simulink library "SUB_ECU_Transmission"  (R2018a)
settings: Solver=VariableStepAuto  StartTime=0.0  StopTime=10.0  RelTol=1e-3
libraries: PTC_MBDS_LIB x38, simulink x9
settings Model: Creator=Sundeep.Tuteja  LastModifiedBy=John.Lahti

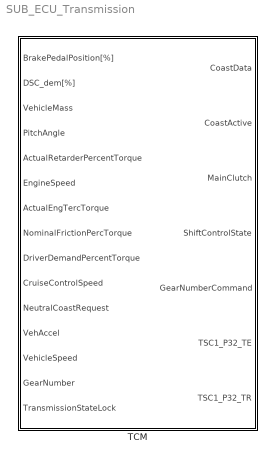
== system SUB_ECU_Transmission ==
  TCM : Subsystem  TreatAsAtomicUnit=on  SystemSampleTime=.01

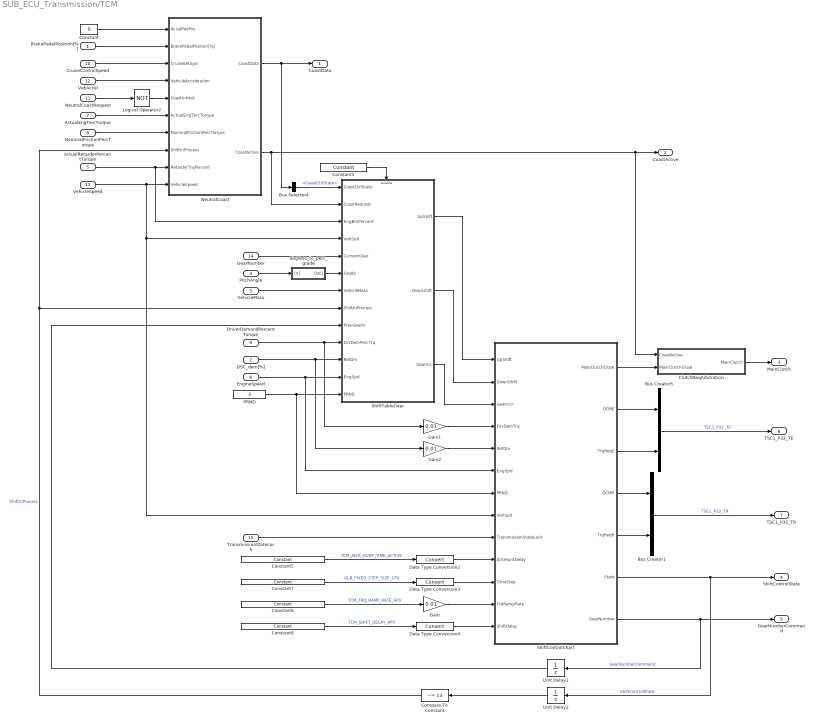
== system SUB_ECU_Transmission/TCM ==
  BrakePedalPosition[%] : Inport  Unit=%
  DSC_dem[%] : Inport  Port=2  Unit=%
  VehicleMass : Inport  Port=3
  PitchAngle : Inport  Port=4
  ActualRetarderPercentTorque : Inport  Port=5
  EngineSpeed : Inport  Port=6
  ActualEngTercTorque : Inport  Port=7
  NominalFrictionPercTorque : Inport  Port=8
  DriverDemandPercentTorque : Inport  Port=9
  CruiseControlSpeed : Inport  Port=10  Unit=km/h
  NeutralCoastRequest : Inport  Port=11
  VehAccel : Inport  Port=12
  VehicleSpeed : Inport  Port=13
  GearNumber : Inport  Port=14
  TransmissionStateLock : Inport  Port=15
  Bus Creator1 : BusCreator  Inputs=2
  Bus Creator5 : BusCreator  Inputs=2
  Bus Selector4 : BusSelector  OutputSignals=CoastCtrlState
  ClutchReqArbitration : Subsystem
  Compare To Constant : simulink/Logic and Bit Operations/Compare To Constant  relop=~=  const=13  OutDataTypeStr=boolean
  Constant : Constant  Value=0
  Constant3 : PTC_MBDS_LIB/Extras/Sources/Constant  Value2=true  PTC_MBDS_BlockVersion=5.41  PTC_BlockType=PTC_MBDS_Constant
      settings: SourceProductName=PACCAR Technical Center MBDS Library
  Constant5 : PTC_MBDS_LIB/Extras/Sources/Constant  Value2=TCM_ANTI_HUNT_TIME_ACTIVE  PTC_MBDS_BlockVersion=5.41  PTC_BlockType=PTC_MBDS_Constant
      settings: SourceProductName=PACCAR Technical Center MBDS Library
      settings: AttributesFormatString=|
      | Value: 1
      | Unit: 's'
  Constant6 : PTC_MBDS_LIB/Extras/Sources/Constant  Value2=TCM_TRQ_RAMP_RATE_APV  PTC_MBDS_BlockVersion=5.41  PTC_BlockType=PTC_MBDS_Constant
      settings: SourceProductName=PACCAR Technical Center MBDS Library
      settings: AttributesFormatString=|
      | Value: 121
      | Unit: '%/s'
  Constant7 : PTC_MBDS_LIB/Extras/Sources/Constant  Value2=GLB_FIXED_STEP_SIZE_CPV  PTC_MBDS_BlockVersion=5.41  PTC_BlockType=PTC_MBDS_Constant
      settings: SourceProductName=PACCAR Technical Center MBDS Library
      settings: AttributesFormatString=|
      | Value: 0.01
      | Unit: 's'
  Constant8 : PTC_MBDS_LIB/Extras/Sources/Constant  Value2=TCM_SHIFT_DELAY_APV  PTC_MBDS_BlockVersion=5.41  PTC_BlockType=PTC_MBDS_Constant
      settings: SourceProductName=PACCAR Technical Center MBDS Library
      settings: AttributesFormatString=|
      | Value: 0.949999988079
      | Unit: 's'
  Data Type Conversion2 : DataTypeConversion  SaturateOnIntegerOverflow=on
  Data Type Conversion3 : DataTypeConversion  SaturateOnIntegerOverflow=on
  Data Type Conversion4 : DataTypeConversion  SaturateOnIntegerOverflow=on
  Gain : Gain  Gain=0.01
  Gain1 : Gain  Gain=0.01
  Gain2 : Gain  Gain=0.01
  Logical Operator2 : Logic  Operator=NOT  AllPortsSameDT=off  OutDataTypeStr=boolean
  NeutralCoast : Subsystem
  PRND : Constant  Value=3
  ShiftControlChart : Stateflow chart  TreatAsAtomicUnit=on
      settings: MinAlgLoopOccurrences=on
  ShiftTableGear : Subsystem
  Unit Delay1 : UnitDelay  SampleTime=-1
  Unit Delay2 : UnitDelay  SampleTime=-1
  degrees_to_perc_grade : Subsystem
  CoastData : Outport
  CoastActive : Outport  Port=2
  MainClutch : Outport  Port=3
  ShiftControlState : Outport  Port=4
  GearNumberCommand : Outport  Port=5
  TSC1_P32_TE : Outport  Port=6
  TSC1_P32_TR : Outport  Port=7
  wires:
  ShiftControlChart/6(State) -> Unit Delay2/1, ShiftControlState/1  "ShiftControlState"
  ShiftControlChart/7(GearNumber) -> Unit Delay1/1, GearNumberCommand/1  "GearNumberCommand"
  Data Type Conversion4/1 -> ShiftControlChart/13(ShiftDelay)
  Data Type Conversion3/1 -> ShiftControlChart/11(TimeStep)
  Data Type Conversion2/1 -> ShiftControlChart/10(AntiHuntDelay)
  VehicleMass/1 -> ShiftTableGear/7(VehicleMass)
  Gain/1 -> ShiftControlChart/12(TrqRampRate)
  Constant3/1 -> ShiftTableGear/Enable
  DSC_dem[%]/1 -> Gain2/1, ShiftTableGear/11(RetDrv)
  Constant8/1 -> Data Type Conversion4/1  "TCM_SHIFT_DELAY_APV"
  Constant6/1 -> Gain/1  "TCM_TRQ_RAMP_RATE_APV"
  VehAccel/1 -> NeutralCoast/4(VehicleAcceleration)
  NeutralCoast/2(CoastActive) -> CoastActive/1, ClutchReqArbitration/1(CoastActive), ShiftTableGear/2(CoastRequest)
  Bus Selector4/1 -> ShiftTableGear/1(CoastCtrlState)  "<CoastCtrlState>"
  ShiftControlChart/1(MainClutchClose) -> ClutchReqArbitration/2(MainClutchClose)
  CruiseControlSpeed/1 -> NeutralCoast/3(CruiseSetSpd)
  Constant5/1 -> Data Type Conversion2/1  "TCM_ANTI_HUNT_TIME_ACTIVE"
  Constant7/1 -> Data Type Conversion3/1  "GLB_FIXED_STEP_SIZE_CPV"
  ClutchReqArbitration/1(MainClutch) -> MainClutch/1
  Constant/1 -> NeutralCoast/1(AccelPedPos)
  VehicleSpeed/1 -> NeutralCoast/10(VehicleSpeed), ShiftControlChart/8(VehSpd), ShiftTableGear/4(VehSpd)
  EngineSpeed/1 -> ShiftTableGear/12(EngSpd), ShiftControlChart/6(EngSpd)
  degrees_to_perc_grade/1(Out1) -> ShiftTableGear/6(Grade)
  TransmissionStateLock/1 -> ShiftControlChart/9(TransmissionStateLock)
  ActualRetarderPercentTorque/1 -> ShiftTableGear/3(EngBrkPercent), NeutralCoast/9(RetarderTrqPercent)
  ActualEngTercTorque/1 -> NeutralCoast/6(ActualEngTercTorque)
  NominalFrictionPercTorque/1 -> NeutralCoast/7(NominalFrictionPercTorque)
  NeutralCoastRequest/1 -> Logical Operator2/1
  ShiftTableGear/1(UpShift) -> ShiftControlChart/1(UpShift)
  ShiftTableGear/2(Downshift) -> ShiftControlChart/2(DownShift)
  ShiftTableGear/3(GearInc) -> ShiftControlChart/3(GearIncr)
  Bus Creator5/1 -> TSC1_P32_TE/1  "TSC1_P32_TE"
  Bus Creator1/1 -> TSC1_P32_TR/1  "TSC1_P32_TR"
  Gain1/1 -> ShiftControlChart/4(DrvDemTrq)
  Gain2/1 -> ShiftControlChart/5(RetDrv)
  ShiftControlChart/2(OCME) -> Bus Creator5/1
  ShiftControlChart/3(TrqReqE) -> Bus Creator5/2
  ShiftControlChart/5(TrqReqR) -> Bus Creator1/2
  ShiftControlChart/4(OCMR) -> Bus Creator1/1
  PRND/1 -> ShiftTableGear/13(PRND), ShiftControlChart/7(PRND)
  Logical Operator2/1 -> NeutralCoast/5(CoastInhibit)
  DriverDemandPercentTorque/1 -> Gain1/1, ShiftTableGear/10(DrvDemPercTrq)
  PitchAngle/1 -> degrees_to_perc_grade/1(In1)
  GearNumber/1 -> ShiftTableGear/5(CurrentGear)
  NeutralCoast/1(CoastData) -> Bus Selector4/1, CoastData/1
  Unit Delay1/1 -> ShiftTableGear/9(PrevGearIn)
  Unit Delay2/1 -> Compare To Constant/1
  Compare To Constant/1 -> NeutralCoast/8(ShiftInProcess), ShiftTableGear/8(ShiftInProcess)  "ShiftInProcess"
  BrakePedalPosition[%]/1 -> NeutralCoast/2(BrakePedalPosition[%])

== system SUB_ECU_Transmission/TCM/ClutchReqArbitration ==
  CoastActive : Inport
  MainClutchClose : Inport  Port=2
  Constant9 : PTC_MBDS_LIB/Extras/Sources/Constant  Value2=TCM_COAST_ENABLE_APV  PTC_MBDS_BlockVersion=5.41  PTC_BlockType=PTC_MBDS_Constant
      settings: SourceProductName=PACCAR Technical Center MBDS Library
      settings: AttributesFormatString=|
      | Value: 1
      | Unit: '1'
  Logical Operator : Logic  AllPortsSameDT=off  OutDataTypeStr=boolean
  Logical Operator1 : Logic  Operator=NAND  AllPortsSameDT=off  OutDataTypeStr=boolean
  MainClutch : Outport
  wires:
  MainClutchClose/1 -> Logical Operator/1
  Logical Operator/1 -> MainClutch/1  "MainClutch"
  CoastActive/1 -> Logical Operator1/1
  Logical Operator1/1 -> Logical Operator/2
  Constant9/1 -> Logical Operator1/2  "TCM_COAST_ENABLE_APV"

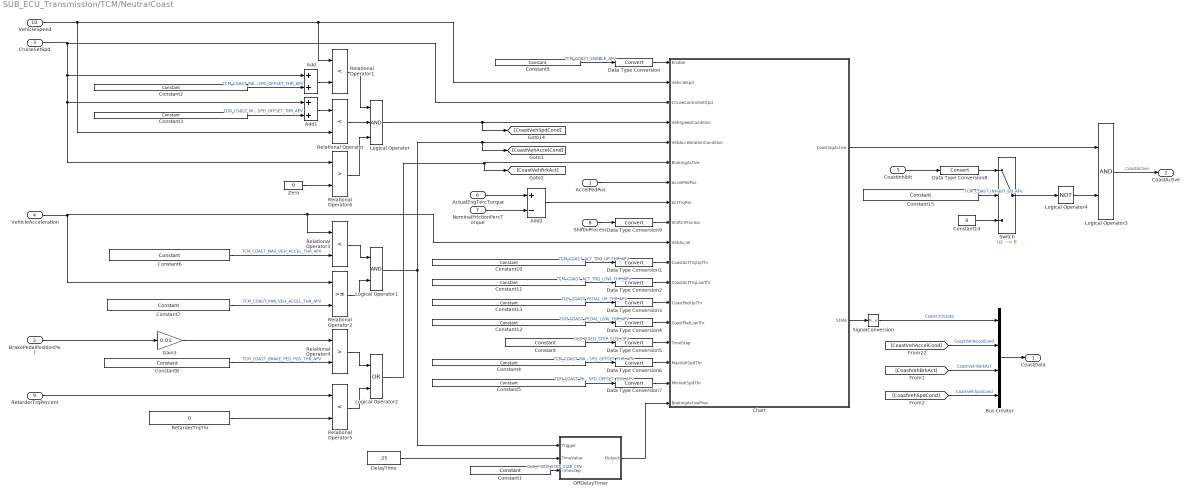
== system SUB_ECU_Transmission/TCM/NeutralCoast ==
  AccelPedPos : Inport
  BrakePedalPosition[%] : Inport  Port=2  Unit=%
  CruiseSetSpd : Inport  Port=3
  VehicleAcceleration : Inport  Port=4
  CoastInhibit : Inport  Port=5
  ActualEngTercTorque : Inport  Port=6
  NominalFrictionPercTorque : Inport  Port=7
  ShiftInProcess : Inport  Port=8
  RetarderTrqPercent : Inport  Port=9
  VehicleSpeed : Inport  Port=10
  Add : Sum
  Add1 : Sum
  Add2 : Sum  Inputs=+-
  Bus Creator : BusCreator  Inputs=4
  Chart : Stateflow chart  TreatAsAtomicUnit=on
  Constant : PTC_MBDS_LIB/Extras/Sources/Constant  Value2=GLB_FIXED_STEP_SIZE_CPV  PTC_MBDS_BlockVersion=5.41  PTC_BlockType=PTC_MBDS_Constant
      settings: SourceProductName=PACCAR Technical Center MBDS Library
      settings: AttributesFormatString=|
      | Value: 0.01
      | Unit: 's'
  Constant1 : PTC_MBDS_LIB/Extras/Sources/Constant  Value2=GLB_FIXED_STEP_SIZE_CPV  PTC_MBDS_BlockVersion=5.41  PTC_BlockType=PTC_MBDS_Constant
      settings: SourceProductName=PACCAR Technical Center MBDS Library
      settings: AttributesFormatString=|
      | Value: 0.01
      | Unit: 's'
  Constant10 : PTC_MBDS_LIB/Extras/Sources/Constant  Value2=TCM_COAST_ACT_TRQ_UP_THR_APV  PTC_MBDS_BlockVersion=5.41  PTC_BlockType=PTC_MBDS_Constant
      settings: SourceProductName=PACCAR Technical Center MBDS Library
      settings: AttributesFormatString=|
      | Value: 20
      | Unit: '%'
  Constant11 : PTC_MBDS_LIB/Extras/Sources/Constant  Value2=TCM_COAST_ACT_TRQ_LOW_THR_APV  PTC_MBDS_BlockVersion=5.41  PTC_BlockType=PTC_MBDS_Constant
      settings: SourceProductName=PACCAR Technical Center MBDS Library
      settings: AttributesFormatString=|
      | Value: 2
      | Unit: '%'
  Constant12 : PTC_MBDS_LIB/Extras/Sources/Constant  Value2=TCM_COAST_PEDAL_LOW_THR_APV  PTC_MBDS_BlockVersion=5.41  PTC_BlockType=PTC_MBDS_Constant
      settings: SourceProductName=PACCAR Technical Center MBDS Library
      settings: AttributesFormatString=|
      | Value: 0
      | Unit: '%'
  Constant13 : PTC_MBDS_LIB/Extras/Sources/Constant  Value2=TCM_COAST_PEDAL_UP_THR_APV  PTC_MBDS_BlockVersion=5.41  PTC_BlockType=PTC_MBDS_Constant
      settings: SourceProductName=PACCAR Technical Center MBDS Library
      settings: AttributesFormatString=|
      | Value: 40
      | Unit: '%'
  Constant14 : Constant  Value=0  OutDataTypeStr=boolean
  Constant15 : PTC_MBDS_LIB/Extras/Sources/Constant  Value2=TCM_COAST_INHIBIT_EN_APV  PTC_MBDS_BlockVersion=5.41  PTC_BlockType=PTC_MBDS_Constant
      settings: SourceProductName=PACCAR Technical Center MBDS Library
      settings: AttributesFormatString=|
      | Value: 1
      | Unit: '1'
  Constant2 : PTC_MBDS_LIB/Extras/Sources/Constant  Value2=TCM_COAST_MAX_VEH_SPD_OFFSET_THR_APV  PTC_MBDS_BlockVersion=5.41  PTC_BlockType=PTC_MBDS_Constant
      settings: SourceProductName=PACCAR Technical Center MBDS Library
      settings: AttributesFormatString=|
      | Value: 10
      | Unit: 'km/h'
  Constant3 : PTC_MBDS_LIB/Extras/Sources/Constant  Value2=TCM_COAST_MIN_VEH_SPD_OFFSET_THR_APV  PTC_MBDS_BlockVersion=5.41  PTC_BlockType=PTC_MBDS_Constant
      settings: SourceProductName=PACCAR Technical Center MBDS Library
      settings: AttributesFormatString=|
      | Value: -10
      | Unit: 'km/h'
  Constant4 : PTC_MBDS_LIB/Extras/Sources/Constant  Value2=TCM_COAST_MAX_VEH_SPD_OFFSET_THR_APV  PTC_MBDS_BlockVersion=5.41  PTC_BlockType=PTC_MBDS_Constant
      settings: SourceProductName=PACCAR Technical Center MBDS Library
      settings: AttributesFormatString=|
      | Value: 10
      | Unit: 'km/h'
  Constant5 : PTC_MBDS_LIB/Extras/Sources/Constant  Value2=TCM_COAST_MIN_VEH_SPD_OFFSET_THR_APV  PTC_MBDS_BlockVersion=5.41  PTC_BlockType=PTC_MBDS_Constant
      settings: SourceProductName=PACCAR Technical Center MBDS Library
      settings: AttributesFormatString=|
      | Value: -10
      | Unit: 'km/h'
  Constant6 : PTC_MBDS_LIB/Extras/Sources/Constant  Value2=TCM_COAST_MAX_VEH_ACCEL_THR_APV  PTC_MBDS_BlockVersion=5.41  PTC_BlockType=PTC_MBDS_Constant
      settings: SourceProductName=PACCAR Technical Center MBDS Library
      settings: AttributesFormatString=|
      | Value: 0.5
      | Unit: 'm/s^2'
  Constant7 : PTC_MBDS_LIB/Extras/Sources/Constant  Value2=TCM_COAST_MIN_VEH_ACCEL_THR_APV  PTC_MBDS_BlockVersion=5.41  PTC_BlockType=PTC_MBDS_Constant
      settings: SourceProductName=PACCAR Technical Center MBDS Library
      settings: AttributesFormatString=|
      | Value: -0.5
      | Unit: 'm/s^2'
  Constant8 : PTC_MBDS_LIB/Extras/Sources/Constant  Value2=TCM_COAST_BRAKE_PED_POS_THR_APV  PTC_MBDS_BlockVersion=5.41  PTC_BlockType=PTC_MBDS_Constant
      settings: SourceProductName=PACCAR Technical Center MBDS Library
      settings: AttributesFormatString=|
      | Value: 0
      | Unit: '1'
  Constant9 : PTC_MBDS_LIB/Extras/Sources/Constant  Value2=TCM_COAST_ENABLE_APV  PTC_MBDS_BlockVersion=5.41  PTC_BlockType=PTC_MBDS_Constant
      settings: SourceProductName=PACCAR Technical Center MBDS Library
      settings: AttributesFormatString=|
      | Value: 1
      | Unit: '1'
  Data Type Conversion{,1..9} (10 alike) : DataTypeConversion  SaturateOnIntegerOverflow=on
  DelayTime : Constant  Value=.25
  Gain3 : Gain  Gain=0.01
  Logical Operator : Logic  Inputs=3  AllPortsSameDT=off  OutDataTypeStr=boolean
  Logical Operator1 : Logic  AllPortsSameDT=off  OutDataTypeStr=boolean
  Logical Operator2 : Logic  Operator=OR  AllPortsSameDT=off  OutDataTypeStr=boolean
  Logical Operator3 : Logic  AllPortsSameDT=off  OutDataTypeStr=boolean
  Logical Operator4 : Logic  Operator=NOT  AllPortsSameDT=off  OutDataTypeStr=boolean
  OffDelayTimer : Subsystem
  Relational Operator{,1,3,5} (4 alike) : RelationalOperator  Operator=<  OutDataTypeStr=boolean  RndMeth=Nearest
  Relational Operator2 : RelationalOperator  OutDataTypeStr=boolean  RndMeth=Nearest
  Relational Operator4 : RelationalOperator  Operator=>  OutDataTypeStr=boolean  RndMeth=Nearest
  Relational Operator6 : RelationalOperator  Operator=>  OutDataTypeStr=boolean  RndMeth=Nearest
  RetarderTrqThr : Constant  Value=0
  SignalConversion : SignalConversion  ConversionOutput=Contiguous copy  OverrideOpt=off
  Switch : Switch  Criteria=u2 ~= 0
  Zero : Constant  Value=0
  CoastData : Outport
  CoastActive : Outport  Port=2
  wires:
  SignalConversion/1 -> Bus Creator/1  "CoastCtrlState"
  Data Type Conversion7/1 -> Chart/17(MinVehSpdThr)
  Data Type Conversion6/1 -> Chart/16(MaxVehSpdThr)
  Data Type Conversion5/1 -> Chart/15(TimeStep)
  Data Type Conversion4/1 -> Chart/14(CoastPedLowThr)
  Data Type Conversion3/1 -> Chart/13(CoastPedUpThr)
  Data Type Conversion2/1 -> Chart/12(CoastActTrqLowThr)
  Data Type Conversion1/1 -> Chart/11(CoastActTrqUpThr)
  Data Type Conversion/1 -> Chart/1(Enable)
  OffDelayTimer/1(Output) -> Chart/18(BrakingActivePrev)
  DelayTime/1 -> OffDelayTimer/2(TimeValue)
  Constant1/1 -> OffDelayTimer/3(TimeStep)  "GLB_FIXED_STEP_SIZE_CPV"
  Constant5/1 -> Data Type Conversion7/1  "TCM_COAST_MIN_VEH_SPD_OFFSET_THR_APV"
  Constant4/1 -> Data Type Conversion6/1  "TCM_COAST_MAX_VEH_SPD_OFFSET_THR_APV"
  Relational Operator6/1 -> Logical Operator/3
  Zero/1 -> Relational Operator6/2
  [CoastVehSpdCond] -> Bus Creator/4  "CoastVehSpdCond"
  [CoastVehBrkAct] -> Bus Creator/3  "CoastVehVBrkAct"
  [CoastVehAccelCond] -> Bus Creator/2  "CoastVehAccelCond"
  Chart/2(State) -> SignalConversion/1
  Bus Creator/1 -> CoastData/1
  VehicleAcceleration/1 -> Relational Operator2/1, Relational Operator3/1, Chart/10(VehAccel)
  VehicleSpeed/1 -> Relational Operator/2, Relational Operator1/1, Chart/2(VehicleSpd)
  CruiseSetSpd/1 -> Add1/1, Relational Operator6/1, Add/1, Chart/3(CruiseControlSetSpd)
  Constant3/1 -> Add1/2  "TCM_COAST_MIN_VEH_SPD_OFFSET_THR_APV"
  Constant2/1 -> Add/2  "TCM_COAST_MAX_VEH_SPD_OFFSET_THR_APV"
  Add/1 -> Relational Operator1/2
  Add1/1 -> Relational Operator/1
  ShiftInProcess/1 -> Data Type Conversion9/1
  Logical Operator2/1 -> [CoastVehBrkAct], Chart/6(BrakingActive)
  Relational Operator5/1 -> Logical Operator2/2
  Relational Operator4/1 -> Logical Operator2/1
  RetarderTrqThr/1 -> Relational Operator5/2
  RetarderTrqPercent/1 -> Relational Operator5/1
  Constant/1 -> Data Type Conversion5/1  "GLB_FIXED_STEP_SIZE_CPV"
  Constant10/1 -> Data Type Conversion1/1  "TCM_COAST_ACT_TRQ_UP_THR_APV"
  Constant11/1 -> Data Type Conversion2/1  "TCM_COAST_ACT_TRQ_LOW_THR_APV"
  Constant13/1 -> Data Type Conversion3/1  "TCM_COAST_PEDAL_UP_THR_APV"
  Constant12/1 -> Data Type Conversion4/1  "TCM_COAST_PEDAL_LOW_THR_APV"
  Constant8/1 -> Relational Operator4/2  "TCM_COAST_BRAKE_PED_POS_THR_APV"
  Add2/1 -> Chart/8(ActTrqPer)
  Relational Operator2/1 -> Logical Operator1/2
  Relational Operator3/1 -> Logical Operator1/1
  Constant7/1 -> Relational Operator2/2  "TCM_COAST_MIN_VEH_ACCEL_THR_APV"
  Constant6/1 -> Relational Operator3/2  "TCM_COAST_MAX_VEH_ACCEL_THR_APV"
  Logical Operator/1 -> Chart/4(VehSpeedCondition), [CoastVehSpdCond]
  Relational Operator/1 -> Logical Operator/2
  Relational Operator1/1 -> Logical Operator/1
  Constant9/1 -> Data Type Conversion/1  "TCM_COAST_ENABLE_APV"
  AccelPedPos/1 -> Chart/7(AccelPedPos)
  Chart/1(CoastingActive) -> Logical Operator3/1
  Logical Operator4/1 -> Logical Operator3/2
  Logical Operator3/1 -> CoastActive/1  "CoastActive"
  Data Type Conversion8/1 -> Switch/1
  Switch/1 -> Logical Operator4/1
  Constant14/1 -> Switch/3
  Constant15/1 -> Switch/2  "TCM_COAST_INHIBIT_EN_APV"
  CoastInhibit/1 -> Data Type Conversion8/1
  Data Type Conversion9/1 -> Chart/9(ShiftInProcess)
  NominalFrictionPercTorque/1 -> Add2/2
  ActualEngTercTorque/1 -> Add2/1
  BrakePedalPosition[%]/1 -> Gain3/1
  Gain3/1 -> Relational Operator4/1
  Logical Operator1/1 -> Chart/5(VehAccelerationCondition), [CoastVehAccelCond], OffDelayTimer/1(Trigger)

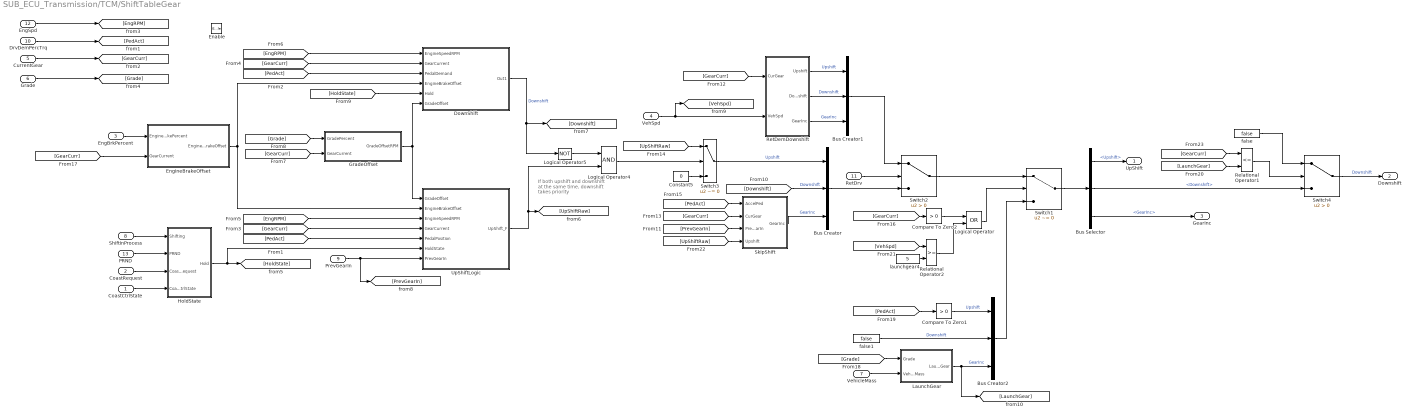
== system SUB_ECU_Transmission/TCM/ShiftTableGear ==
  note: If both upshift and
      | downshift at the same
      | time, downshift takes
      | priority
  CoastCtrlState : Inport
  CoastRequest : Inport  Port=2
  EngBrkPercent : Inport  Port=3
  VehSpd : Inport  Port=4
  CurrentGear : Inport  Port=5
  Grade : Inport  Port=6
  VehicleMass : Inport  Port=7
  ShiftInProcess : Inport  Port=8
  PrevGearIn : Inport  Port=9
  DrvDemPercTrq : Inport  Port=10  Unit=%
  RetDrv : Inport  Port=11
  EngSpd : Inport  Port=12
  PRND : Inport  Port=13
  Enable : EnablePort  PropagateVarSize=During execution
  Bus Creator : BusCreator  Inputs=3
  Bus Creator1 : BusCreator  Inputs=3
  Bus Creator2 : BusCreator  Inputs=3
  Bus Selector : BusSelector  OutputSignals=Upshift,Downshift,GearInc
  Compare To Zero1 : simulink/Logic and Bit Operations/Compare To Zero  relop=>  OutDataTypeStr=boolean
  Compare To Zero2 : simulink/Logic and Bit Operations/Compare To Zero  relop=>  OutDataTypeStr=boolean
  Constant5 : Constant  Value=0  OutDataTypeStr=boolean
  DownShift : Subsystem
  EngineBrakeOffset : Subsystem
  GradeOffset : Subsystem
  HoldState : Subsystem
  LaunchGear : Subsystem
  Logical Operator : Logic  Operator=OR  AllPortsSameDT=off  OutDataTypeStr=boolean
  Logical Operator4 : Logic  AllPortsSameDT=off  OutDataTypeStr=boolean
  Logical Operator5 : Logic  Operator=NOT  AllPortsSameDT=off  OutDataTypeStr=boolean
  Relational Operator1 : RelationalOperator  Operator=<=  OutDataTypeStr=boolean  RndMeth=Nearest
  Relational Operator2 : RelationalOperator  OutDataTypeStr=boolean  RndMeth=Nearest
  RetDemDownshift : Subsystem
  SkipShift : Subsystem
  Switch1 : Switch  Criteria=u2 ~= 0
  Switch2 : Switch  Criteria=u2 > Threshold
  Switch3 : Switch  Criteria=u2 ~= 0
  Switch4 : Switch  Criteria=u2 > Threshold
  UpShiftLogic : Subsystem
  false : Constant  Value=false  OutDataTypeStr=boolean
  false1 : Constant  Value=false  OutDataTypeStr=boolean
  launchgear4 : Constant  Value=5
  UpShift : Outport
  Downshift : Outport  Port=2
  GearInc : Outport  Port=3
  wires:
  VehicleMass/1 -> LaunchGear/2(VehicleMass)
  Compare To Zero2/1 -> Logical Operator/1
  Logical Operator/1 -> Switch1/2
  [GearCurr] -> Compare To Zero2/1
  Relational Operator2/1 -> Logical Operator/2
  [VehSpd] -> Relational Operator2/1
  launchgear4/1 -> Relational Operator2/2
  Relational Operator1/1 -> Switch4/2
  [LaunchGear] -> Relational Operator1/2
  [PedAct] -> Compare To Zero1/1
  [UpShiftRaw] -> SkipShift/4(Upshift)
  false/1 -> Switch4/1
  Switch4/1 -> Downshift/1  "Downshift"
  [GearCurr] -> Relational Operator1/1
  Bus Creator2/1 -> Switch1/3
  LaunchGear/1(LaunchGear) -> Bus Creator2/3, [LaunchGear]  "GearInc"
  false1/1 -> Bus Creator2/2  "Downshift"
  Compare To Zero1/1 -> Bus Creator2/1  "Upshift"
  [Grade] -> LaunchGear/1(Grade)
  Switch2/1 -> Switch1/1
  Switch1/1 -> Bus Selector/1
  Bus Selector/1 -> UpShift/1  "<Upshift>"
  Bus Selector/2 -> Switch4/3  "<Downshift>"
  Bus Selector/3 -> GearInc/1  "<GearInc>"
  SkipShift/1(GearInc) -> Bus Creator/3  "GearInc"
  [PrevGearIn] -> SkipShift/3(PrevGearIn)
  [GearCurr] -> SkipShift/2(CurGear)
  RetDemDownshift/3(GearInc) -> Bus Creator1/3  "GearInc"
  RetDemDownshift/2(Downshift) -> Bus Creator1/2  "Downshift"
  RetDemDownshift/1(Upshift) -> Bus Creator1/1  "Upshift"
  VehSpd/1 -> RetDemDownshift/2(VehSpd), [VehSpd]
  [GearCurr] -> RetDemDownshift/1(CurGear)
  Bus Creator1/1 -> Switch2/1
  [Downshift] -> Bus Creator/2  "Downshift"
  Bus Creator/1 -> Switch2/3
  Switch3/1 -> Bus Creator/1  "Upshift"
  RetDrv/1 -> Switch2/2
  CoastCtrlState/1 -> HoldState/4(CoastCtrlState)
  CoastRequest/1 -> HoldState/3(CoastRequest)
  [HoldState] -> DownShift/5(Hold)
  PRND/1 -> HoldState/2(PRND)
  ShiftInProcess/1 -> HoldState/1(Shifting)
  GradeOffset/1(GradeOffsetRPM) -> DownShift/6(GradeOffset), UpShiftLogic/1(GradeOffset)
  [GearCurr] -> EngineBrakeOffset/2(GearCurrent)
  EngBrkPercent/1 -> EngineBrakeOffset/1(EngineBrakePercent)
  EngineBrakeOffset/1(EngineBrakeOffset) -> DownShift/4(EngineBrakeOffset), UpShiftLogic/2(EngineBrakeOffset)
  [PedAct] -> DownShift/3(PedalDemand)
  [GearCurr] -> DownShift/2(GearCurrent)
  [EngRPM] -> DownShift/1(EngineSpeedRPM)
  DownShift/1(Out1) -> Logical Operator5/1, [Downshift]  "Downshift"
  PrevGearIn/1 -> [PrevGearIn], UpShiftLogic/7(PrevGearIn)
  HoldState/1(Hold) -> UpShiftLogic/6(HoldState), [HoldState]
  [PedAct] -> UpShiftLogic/5(PedalPosition)
  [GearCurr] -> UpShiftLogic/4(GearCurrent)
  [EngRPM] -> UpShiftLogic/3(EngineSpeedRPM)
  UpShiftLogic/1(UpShift_F) -> [UpShiftRaw], Logical Operator4/2
  [GearCurr] -> GradeOffset/2(GearCurrent)
  [Grade] -> GradeOffset/1(GradePercent)
  DrvDemPercTrq/1 -> [PedAct]
  [UpShiftRaw] -> Switch3/1
  Logical Operator5/1 -> Logical Operator4/1
  Grade/1 -> [Grade]
  EngSpd/1 -> [EngRPM]
  Constant5/1 -> Switch3/3
  Logical Operator4/1 -> Switch3/2
  CurrentGear/1 -> [GearCurr]
  [PedAct] -> SkipShift/1(AccelPed)

== system SUB_ECU_Transmission/TCM/degrees_to_perc_grade ==
  In1 : Inport
  Gain : Gain  Gain=pi/180
  Gain1 : Gain  Gain=100
  Trigonometric Function : Trigonometry  Operator=tan
  Out1 : Outport
  wires:
  In1/1 -> Gain/1
  Gain/1 -> Trigonometric Function/1
  Trigonometric Function/1 -> Gain1/1
  Gain1/1 -> Out1/1

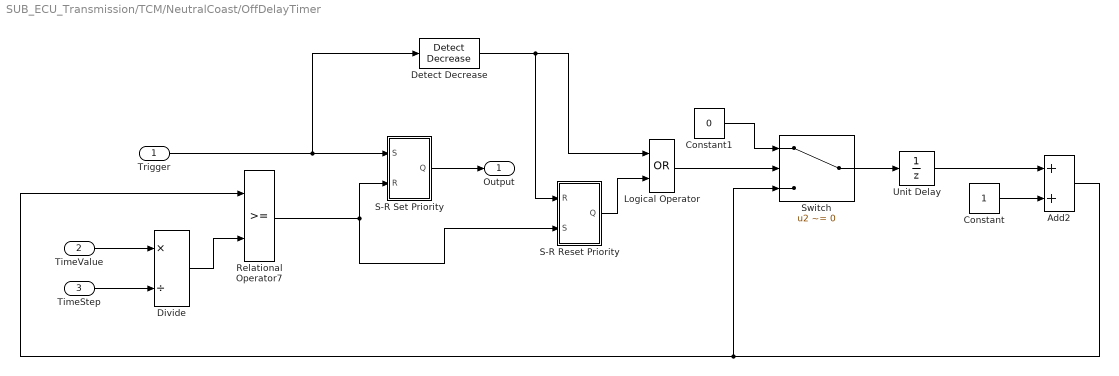
== system SUB_ECU_Transmission/TCM/NeutralCoast/OffDelayTimer ==
  Trigger : Inport
  TimeValue : Inport  Port=2
  TimeStep : Inport  Port=3
  Add2 : Sum
  Constant : Constant
  Constant1 : Constant  Value=0
  Detect Decrease : simulink/Logic and Bit Operations/Detect Decrease  vinit=0.0  OutDataTypeStr=boolean
  Divide : Product  Inputs=*/
  Logical Operator : Logic  Operator=OR  AllPortsSameDT=off  OutDataTypeStr=boolean
  Relational Operator7 : RelationalOperator  OutDataTypeStr=boolean  RndMeth=Nearest
  S-R Reset Priority : Subsystem
  S-R Set Priority : Subsystem
  Switch : Switch  Criteria=u2 ~= 0
  Unit Delay : UnitDelay  SampleTime=-1
  Output : Outport
  wires:
  S-R Reset Priority/1(Q) -> Logical Operator/2
  Logical Operator/1 -> Switch/2
  Relational Operator7/1 -> S-R Reset Priority/2(S), S-R Set Priority/2(R)
  Detect Decrease/1 -> Logical Operator/1, S-R Reset Priority/1(R)
  Divide/1 -> Relational Operator7/2
  TimeStep/1 -> Divide/2
  Constant1/1 -> Switch/1
  Trigger/1 -> S-R Set Priority/1(S), Detect Decrease/1
  TimeValue/1 -> Divide/1
  S-R Set Priority/1(Q) -> Output/1
  Add2/1 -> Relational Operator7/1, Switch/3
  Constant/1 -> Add2/2
  Unit Delay/1 -> Add2/1
  Switch/1 -> Unit Delay/1

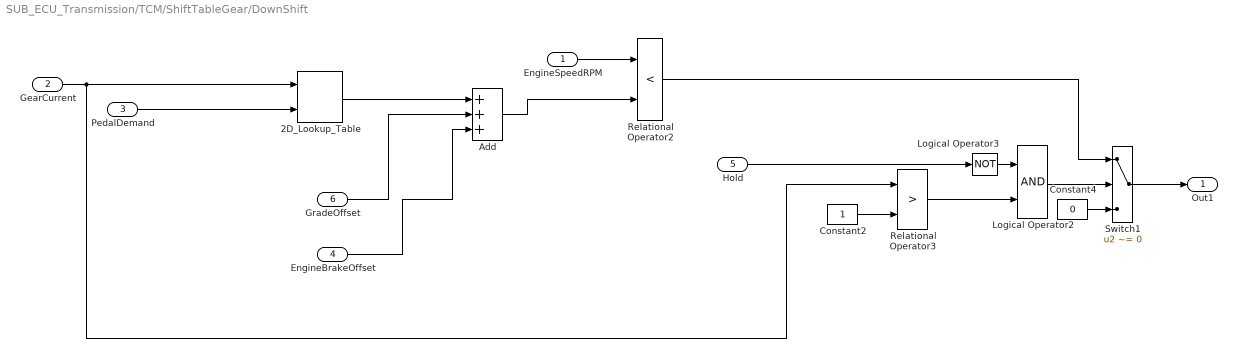
== system SUB_ECU_Transmission/TCM/ShiftTableGear/DownShift ==
  EngineSpeedRPM : Inport
  GearCurrent : Inport  Port=2
  PedalDemand : Inport  Port=3
  EngineBrakeOffset : Inport  Port=4
  Hold : Inport  Port=5
  GradeOffset : Inport  Port=6
  2D_Lookup_Table : PTC_MBDS_LIB/Extras/Lookup Tables/2D_Lookup_Table  ParameterObjectName=TCM_NCRS_SHIFT_DOWN_DATA_MPV  InterpolationMethod=Linear  PTC_MBDS_BlockVersion=5.41  PTC_BlockType=PTC_MBDS_2D_Lookup_Table
      settings: SourceProductName=PACCAR Technical Center MBDS Library
      settings: AttributesFormatString=|
      | Row Axis: TCM_NCRS_SHIFT_DOWN_GEARNUM_STEP_MPV (1)
      | Column Axis: TCM_NCRS_SHIFT_DOWN_THROTTLE_STEP_MPV (%)
      | Data Axis: TCM_NCRS_SHIFT_DOWN_DATA_MPV (rpm)
      | Interpolation Method: Linear
  Add : Sum  Inputs=+++
  Constant2 : Constant
  Constant4 : Constant  Value=0  OutDataTypeStr=boolean
  Logical Operator2 : Logic  AllPortsSameDT=off  OutDataTypeStr=boolean
  Logical Operator3 : Logic  Operator=NOT  AllPortsSameDT=off  OutDataTypeStr=boolean
  Relational Operator2 : RelationalOperator  Operator=<  OutDataTypeStr=boolean  RndMeth=Nearest
  Relational Operator3 : RelationalOperator  Operator=>  OutDataTypeStr=boolean  RndMeth=Nearest
  Switch1 : Switch  Criteria=u2 ~= 0
  Out1 : Outport
  wires:
  EngineBrakeOffset/1 -> Add/3
  GradeOffset/1 -> Add/2
  Add/1 -> Relational Operator2/2
  2D_Lookup_Table/1 -> Add/1
  PedalDemand/1 -> 2D_Lookup_Table/2
  Switch1/1 -> Out1/1
  Relational Operator2/1 -> Switch1/1
  Constant2/1 -> Relational Operator3/2
  GearCurrent/1 -> 2D_Lookup_Table/1, Relational Operator3/1
  Constant4/1 -> Switch1/3
  Logical Operator2/1 -> Switch1/2
  Hold/1 -> Logical Operator3/1
  Relational Operator3/1 -> Logical Operator2/2
  Logical Operator3/1 -> Logical Operator2/1
  EngineSpeedRPM/1 -> Relational Operator2/1

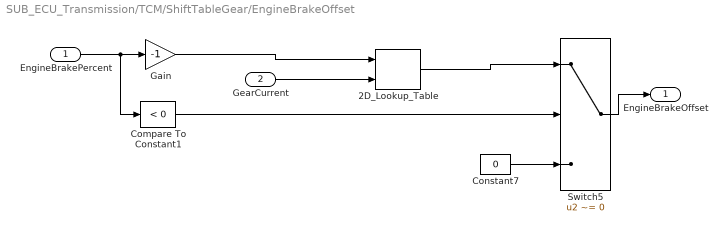
== system SUB_ECU_Transmission/TCM/ShiftTableGear/EngineBrakeOffset ==
  EngineBrakePercent : Inport
  GearCurrent : Inport  Port=2
  2D_Lookup_Table : PTC_MBDS_LIB/Extras/Lookup Tables/2D_Lookup_Table  ParameterObjectName=TCM_SHIFT_ENG_BRAKE_OFFSET_DATA_MPV  InterpolationMethod=Linear  PTC_MBDS_BlockVersion=5.41  PTC_BlockType=PTC_MBDS_2D_Lookup_Table
      settings: SourceProductName=PACCAR Technical Center MBDS Library
      settings: AttributesFormatString=|
      | Row Axis: TCM_SHIFT_ENG_BRAKE_RETARDER_TRQ_MPV (%)
      | Column Axis: TCM_SHIFT_GEAR_NUMBER_MPV (rpm)
      | Data Axis: TCM_SHIFT_ENG_BRAKE_OFFSET_DATA_MPV (rpm)
      | Interpolation Method: Linear
  Compare To Constant1 : simulink/Logic and Bit Operations/Compare To Constant  relop=<  const=0  OutDataTypeStr=boolean
  Constant7 : Constant  Value=0  OutDataTypeStr=boolean
  Gain : Gain  Gain=-1
  Switch5 : Switch  Criteria=u2 ~= 0
  EngineBrakeOffset : Outport
  wires:
  Gain/1 -> 2D_Lookup_Table/1
  Constant7/1 -> Switch5/3
  Compare To Constant1/1 -> Switch5/2
  Switch5/1 -> EngineBrakeOffset/1
  2D_Lookup_Table/1 -> Switch5/1
  EngineBrakePercent/1 -> Compare To Constant1/1, Gain/1
  GearCurrent/1 -> 2D_Lookup_Table/2

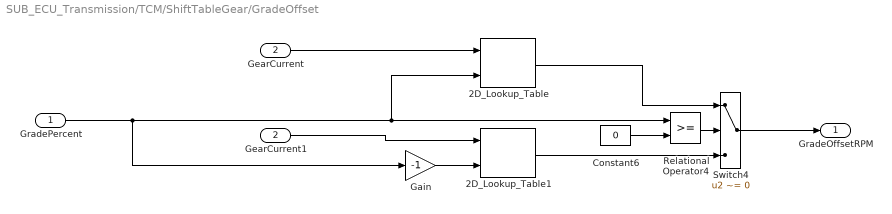
== system SUB_ECU_Transmission/TCM/ShiftTableGear/GradeOffset ==
  GradePercent : Inport
  GearCurrent : Inport  Port=2
  2D_Lookup_Table : PTC_MBDS_LIB/Extras/Lookup Tables/2D_Lookup_Table  ParameterObjectName=TCM_SHIFT_UPGRADE_OFFSET_DATA_MPV  InterpolationMethod=Linear  PTC_MBDS_BlockVersion=5.41  PTC_BlockType=PTC_MBDS_2D_Lookup_Table
      settings: SourceProductName=PACCAR Technical Center MBDS Library
      settings: AttributesFormatString=|
      | Row Axis: TCM_SHIFT_UPGRADE_GEARNUM_STEP_MPV (1)
      | Column Axis: TCM_SHIFT_UPGRADE_GRADEPERC_STEP_MPV (%)
      | Data Axis: TCM_SHIFT_UPGRADE_OFFSET_DATA_MPV (rpm)
      | Interpolation Method: Linear
  2D_Lookup_Table1 : PTC_MBDS_LIB/Extras/Lookup Tables/2D_Lookup_Table  ParameterObjectName=TCM_SHIFT_DOWNGRADE_OFFSET_DATA_MPV  InterpolationMethod=Linear  PTC_MBDS_BlockVersion=5.41  PTC_BlockType=PTC_MBDS_2D_Lookup_Table
      settings: SourceProductName=PACCAR Technical Center MBDS Library
      settings: AttributesFormatString=|
      | Row Axis: TCM_SHIFT_DOWNGRADE_GEARNUM_STEP_MPV (1)
      | Column Axis: TCM_SHIFT_DOWNGRADE_GRADEPERC_STEP_MPV (%)
      | Data Axis: TCM_SHIFT_DOWNGRADE_OFFSET_DATA_MPV (rpm)
      | Interpolation Method: Linear
  Constant6 : Constant  Value=0  OutDataTypeStr=boolean
  Gain : Gain  Gain=-1
  GearCurrent1 : InportShadow  Port=2
  Relational Operator4 : RelationalOperator  OutDataTypeStr=boolean  RndMeth=Nearest
  Switch4 : Switch  Criteria=u2 ~= 0
  GradeOffsetRPM : Outport
  wires:
  Switch4/1 -> GradeOffsetRPM/1
  2D_Lookup_Table1/1 -> Switch4/3
  2D_Lookup_Table/1 -> Switch4/1
  Gain/1 -> 2D_Lookup_Table1/2
  Constant6/1 -> Relational Operator4/2
  GradePercent/1 -> Gain/1, Relational Operator4/1, 2D_Lookup_Table/2
  Relational Operator4/1 -> Switch4/2
  GearCurrent1/1 -> 2D_Lookup_Table1/1
  GearCurrent/1 -> 2D_Lookup_Table/1

== system SUB_ECU_Transmission/TCM/ShiftTableGear/HoldState ==
  Shifting : Inport
  PRND : Inport  Port=2
  CoastRequest : Inport  Port=3
  CoastCtrlState : Inport  Port=4
  Compare To Constant : simulink/Logic and Bit Operations/Compare To Constant  relop=~=  const=3.0  OutDataTypeStr=uint8  ZeroCross=off
  Compare To Constant1 : simulink/Logic and Bit Operations/Compare To Constant  relop===  const=4  OutDataTypeStr=uint8  ZeroCross=off
  Logical Operator : Logic  Operator=OR  Inputs=4  AllPortsSameDT=off  OutDataTypeStr=boolean
  Hold : Outport
  wires:
  Compare To Constant1/1 -> Logical Operator/4
  CoastCtrlState/1 -> Compare To Constant1/1
  CoastRequest/1 -> Logical Operator/3
  Compare To Constant/1 -> Logical Operator/2
  PRND/1 -> Compare To Constant/1
  Logical Operator/1 -> Hold/1
  Shifting/1 -> Logical Operator/1

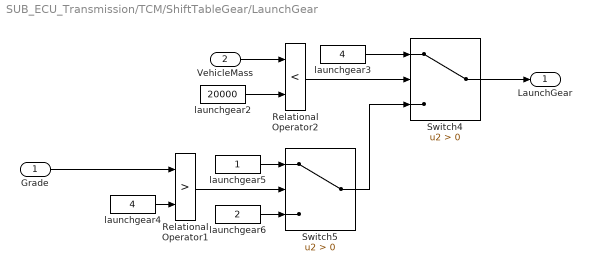
== system SUB_ECU_Transmission/TCM/ShiftTableGear/LaunchGear ==
  Grade : Inport
  VehicleMass : Inport  Port=2
  Relational Operator1 : RelationalOperator  Operator=>  OutDataTypeStr=boolean  RndMeth=Nearest
  Relational Operator2 : RelationalOperator  Operator=<  OutDataTypeStr=boolean  RndMeth=Nearest
  Switch4 : Switch  Criteria=u2 > Threshold
  Switch5 : Switch  Criteria=u2 > Threshold
  launchgear2 : Constant  Value=20000
  launchgear3 : Constant  Value=4
  launchgear4 : Constant  Value=4
  launchgear5 : Constant
  launchgear6 : Constant  Value=2
  LaunchGear : Outport
  wires:
  Switch4/1 -> LaunchGear/1
  launchgear6/1 -> Switch5/3
  launchgear4/1 -> Relational Operator1/2
  launchgear5/1 -> Switch5/1
  Grade/1 -> Relational Operator1/1
  VehicleMass/1 -> Relational Operator2/1
  launchgear3/1 -> Switch4/1
  launchgear2/1 -> Relational Operator2/2
  Relational Operator2/1 -> Switch4/2
  Relational Operator1/1 -> Switch5/2
  Switch5/1 -> Switch4/3

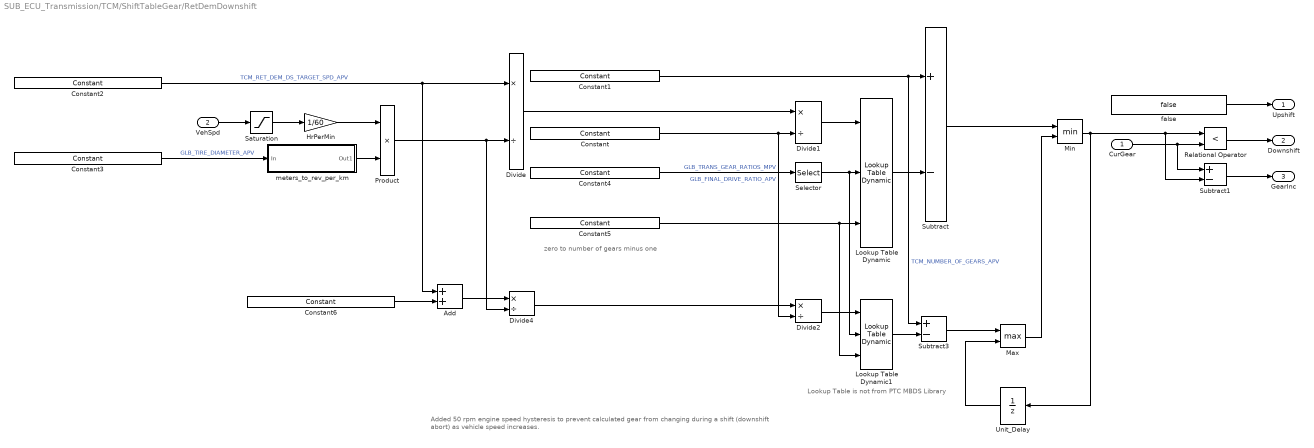
== system SUB_ECU_Transmission/TCM/ShiftTableGear/RetDemDownshift ==
  note: Lookup Table is not from PTC MBDS Library
  note: Added 50 rpm engine speed hysteresis to prevent calculated gear from changing during a shift (downshift abort) as vehicle speed increases.
  note: zero to number of gears minus one
  CurGear : Inport
  VehSpd : Inport  Port=2
  Add : Sum  OutDataTypeStr=Inherit: Inherit via back propagation  SaturateOnIntegerOverflow=on  InputSameDT=on
      settings: AttributesFormatString=Saturate: %<SaturateOnIntegerOverflow>
  Constant : PTC_MBDS_LIB/Extras/Sources/Constant  Value2=GLB_FINAL_DRIVE_RATIO_APV  PTC_MBDS_BlockVersion=5.41  PTC_BlockType=PTC_MBDS_Constant
      settings: SourceProductName=PACCAR Technical Center MBDS Library
      settings: AttributesFormatString=|
      | Value: 2.6400001049
      | Unit: '1'
  Constant1 : PTC_MBDS_LIB/Extras/Sources/Constant  Value2=TCM_NUMBER_OF_GEARS_APV  PTC_MBDS_BlockVersion=5.41  PTC_BlockType=PTC_MBDS_Constant
      settings: SourceProductName=PACCAR Technical Center MBDS Library
      settings: AttributesFormatString=|
      | Value: 12
      | Unit: '1'
  Constant2 : PTC_MBDS_LIB/Extras/Sources/Constant  Value2=TCM_RET_DEM_DS_TARGET_SPD_APV  PTC_MBDS_BlockVersion=5.41  PTC_BlockType=PTC_MBDS_Constant
      settings: SourceProductName=PACCAR Technical Center MBDS Library
      settings: AttributesFormatString=|
      | Value: 1950
      | Unit: 'rpm'
  Constant3 : PTC_MBDS_LIB/Extras/Sources/Constant  Value2=GLB_TIRE_DIAMETER_APV  PTC_MBDS_BlockVersion=5.41  PTC_BlockType=PTC_MBDS_Constant
      settings: SourceProductName=PACCAR Technical Center MBDS Library
      settings: AttributesFormatString=|
      | Value: 1
      | Unit: 'm'
  Constant4 : PTC_MBDS_LIB/Extras/Sources/Constant  Value2=GLB_TRANS_GEAR_RATIOS_MPV  PTC_MBDS_BlockVersion=5.41  PTC_BlockType=PTC_MBDS_Constant
      settings: SourceProductName=PACCAR Technical Center MBDS Library
      settings: AttributesFormatString=|
      | Value: <1 X 12>
      | Unit: '1'
  Constant5 : PTC_MBDS_LIB/Extras/Sources/Constant  Value2=0:11  PTC_MBDS_BlockVersion=5.41  PTC_BlockType=PTC_MBDS_Constant
      settings: SourceProductName=PACCAR Technical Center MBDS Library
  Constant6 : PTC_MBDS_LIB/Extras/Sources/Constant  Value2=50  PTC_MBDS_BlockVersion=5.41  PTC_BlockType=PTC_MBDS_Constant
      settings: SourceProductName=PACCAR Technical Center MBDS Library
  Divide : Product  Inputs=*/
  Divide1 : Product  Inputs=*/
  Divide2 : Product  Inputs=*/  OutDataTypeStr=Inherit: Inherit via back propagation  SaturateOnIntegerOverflow=on  InputSameDT=on
      settings: AttributesFormatString=Saturate: %<SaturateOnIntegerOverflow>
  Divide4 : Product  Inputs=*/  OutDataTypeStr=Inherit: Inherit via back propagation  SaturateOnIntegerOverflow=on  InputSameDT=on
      settings: AttributesFormatString=Saturate: %<SaturateOnIntegerOverflow>
  HrPerMin : Gain  Gain=1/60
  Lookup Table Dynamic : simulink/Lookup Tables/Lookup Table Dynamic  LookUpMeth=Use Input Below  OutDataType=fixdt('double')  OutScaling=[]  OutputDataTypeScalingMode=Specify via dialog  OutDataTypeStr=fixdt('double')  DoSatur=off
      settings: SourceProductName=Simulink
  Lookup Table Dynamic1 : simulink/Lookup Tables/Lookup Table Dynamic  LookUpMeth=Use Input Below  OutDataType=fixdt('double')  OutScaling=[]  OutputDataTypeScalingMode=Specify via dialog  OutDataTypeStr=fixdt('double')  DoSatur=off
      settings: SourceProductName=Simulink
  Max : MinMax  Function=max  Inputs=2  OutDataTypeStr=Inherit: Inherit via back propagation  SaturateOnIntegerOverflow=on  InputSameDT=on
  Min : MinMax  Inputs=2  OutDataTypeStr=Inherit: Inherit via back propagation  SaturateOnIntegerOverflow=on  InputSameDT=on
  Product : Product
  Relational Operator : RelationalOperator  Operator=<  OutDataTypeStr=boolean  RndMeth=Nearest
  Saturation : Saturate  UpperLimit=Inf  LowerLimit=0.1
  Selector : Selector  InputPortWidth=12  IndexOptions=Index vector (dialog)  Indices=12:-1:1  OutputSizes=1
  Subtract : Sum  Inputs=+-
  Subtract1 : Sum  Inputs=+-
  Subtract3 : Sum  Inputs=+-  OutDataTypeStr=Inherit: Inherit via back propagation  SaturateOnIntegerOverflow=on  InputSameDT=on
      settings: AttributesFormatString=Saturate: %<SaturateOnIntegerOverflow>
  Unit_Delay : UnitDelay  SampleTime=-1
      settings: AttributesFormatString=Init = %<InitialCondition>
  false : Constant  Value=false  OutDataTypeStr=boolean
  meters_to_rev_per_km : Subsystem
  Upshift : Outport
  Downshift : Outport  Port=2
  GearInc : Outport  Port=3
  wires:
  Subtract3/1 -> Max/1
  Divide1/1 -> Lookup Table Dynamic/1
  Constant5/1 -> Lookup Table Dynamic1/3, Lookup Table Dynamic/3
  Constant4/1 -> Selector/1  "GLB_TRANS_GEAR_RATIOS_MPV"
  Constant3/1 -> meters_to_rev_per_km/1(In)  "GLB_TIRE_DIAMETER_APV"
  Saturation/1 -> HrPerMin/1
  Min/1 -> Unit_Delay/1, Subtract1/2, Relational Operator/1
  Subtract1/1 -> GearInc/1
  Relational Operator/1 -> Downshift/1
  CurGear/1 -> Relational Operator/2, Subtract1/1
  Constant1/1 -> Subtract3/1, Subtract/1  "TCM_NUMBER_OF_GEARS_APV"
  Divide/1 -> Divide1/1
  Constant/1 -> Divide1/2, Divide2/2  "GLB_FINAL_DRIVE_RATIO_APV"
  Product/1 -> Divide/2, Divide4/2
  Constant2/1 -> Divide/1, Add/1  "TCM_RET_DEM_DS_TARGET_SPD_APV"
  meters_to_rev_per_km/1(Out1) -> Product/2
  HrPerMin/1 -> Product/1
  VehSpd/1 -> Saturation/1
  false/1 -> Upshift/1
  Lookup Table Dynamic/1 -> Subtract/2
  Lookup Table Dynamic1/1 -> Subtract3/2
  Divide4/1 -> Divide2/1
  Selector/1 -> Lookup Table Dynamic1/2, Lookup Table Dynamic/2
  Divide2/1 -> Lookup Table Dynamic1/1
  Constant6/1 -> Add/2
  Add/1 -> Divide4/1
  Subtract/1 -> Min/1
  Max/1 -> Min/2
  Unit_Delay/1 -> Max/2

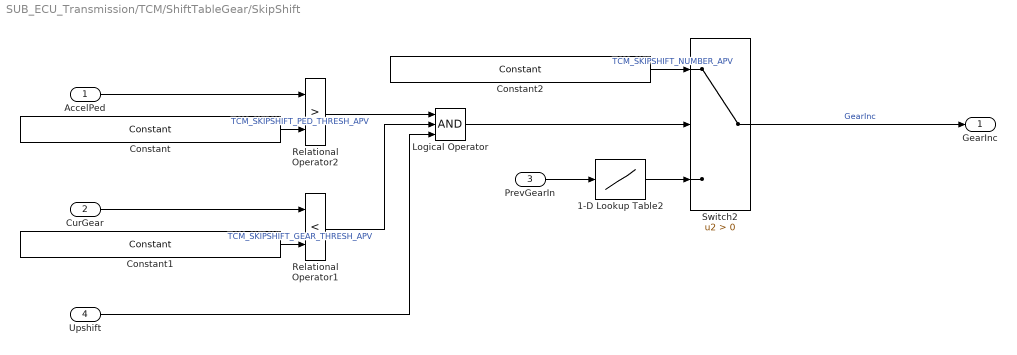
== system SUB_ECU_Transmission/TCM/ShiftTableGear/SkipShift ==
  AccelPed : Inport
  CurGear : Inport  Port=2
  PrevGearIn : Inport  Port=3
  Upshift : Inport  Port=4
  1-D Lookup Table2 : Lookup_n-D  NumberOfTableDimensions=1  BreakpointsForDimension1=[1:1:18]  Table=[1 1 1 1 1 1 1 1 1 1 1 1 1 1 1 1 1 1]  InternalRulePriority=Speed  RndMeth=Simplest  InputSameDT=on
  Constant : PTC_MBDS_LIB/Extras/Sources/Constant  Value2=TCM_SKIPSHIFT_PED_THRESH_APV  PTC_MBDS_BlockVersion=5.41  PTC_BlockType=PTC_MBDS_Constant
      settings: SourceProductName=PACCAR Technical Center MBDS Library
      settings: AttributesFormatString=|
      | Value: 0.300000011921
      | Unit: '%'
  Constant1 : PTC_MBDS_LIB/Extras/Sources/Constant  Value2=TCM_SKIPSHIFT_GEAR_THRESH_APV  PTC_MBDS_BlockVersion=5.41  PTC_BlockType=PTC_MBDS_Constant
      settings: SourceProductName=PACCAR Technical Center MBDS Library
      settings: AttributesFormatString=|
      | Value: 7
      | Unit: '1'
  Constant2 : PTC_MBDS_LIB/Extras/Sources/Constant  Value2=TCM_SKIPSHIFT_NUMBER_APV  PTC_MBDS_BlockVersion=5.41  PTC_BlockType=PTC_MBDS_Constant
      settings: SourceProductName=PACCAR Technical Center MBDS Library
      settings: AttributesFormatString=|
      | Value: 2
      | Unit: '1'
  Logical Operator : Logic  Inputs=3  AllPortsSameDT=off  OutDataTypeStr=boolean
  Relational Operator1 : RelationalOperator  Operator=<  OutDataTypeStr=boolean  RndMeth=Nearest
  Relational Operator2 : RelationalOperator  Operator=>  OutDataTypeStr=boolean  RndMeth=Nearest
  Switch2 : Switch  Criteria=u2 > Threshold
  GearInc : Outport
  wires:
  Upshift/1 -> Logical Operator/3
  1-D Lookup Table2/1 -> Switch2/3
  PrevGearIn/1 -> 1-D Lookup Table2/1
  Constant2/1 -> Switch2/1  "TCM_SKIPSHIFT_NUMBER_APV"
  Relational Operator1/1 -> Logical Operator/2
  Relational Operator2/1 -> Logical Operator/1
  Logical Operator/1 -> Switch2/2
  Switch2/1 -> GearInc/1  "GearInc"
  AccelPed/1 -> Relational Operator2/1
  Constant/1 -> Relational Operator2/2  "TCM_SKIPSHIFT_PED_THRESH_APV"
  CurGear/1 -> Relational Operator1/1
  Constant1/1 -> Relational Operator1/2  "TCM_SKIPSHIFT_GEAR_THRESH_APV"

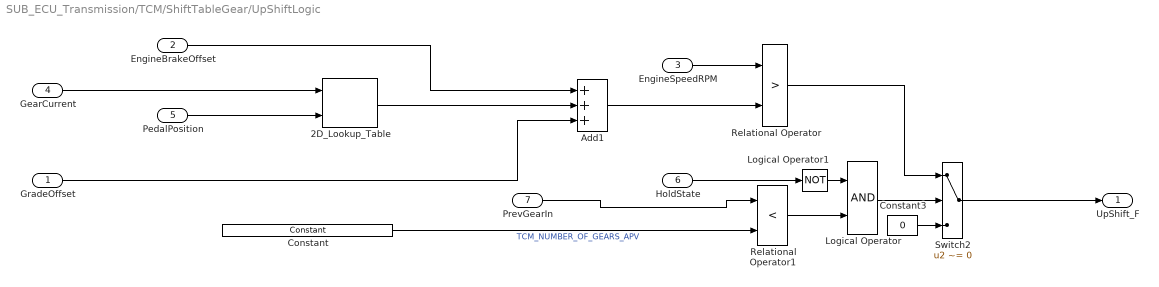
== system SUB_ECU_Transmission/TCM/ShiftTableGear/UpShiftLogic ==
  GradeOffset : Inport
  EngineBrakeOffset : Inport  Port=2
  EngineSpeedRPM : Inport  Port=3
  GearCurrent : Inport  Port=4
  PedalPosition : Inport  Port=5
  HoldState : Inport  Port=6
  PrevGearIn : Inport  Port=7
  2D_Lookup_Table : PTC_MBDS_LIB/Extras/Lookup Tables/2D_Lookup_Table  ParameterObjectName=TCM_NCRS_SHIFT_UP_DATA_MPV  InterpolationMethod=Linear  PTC_MBDS_BlockVersion=5.41  PTC_BlockType=PTC_MBDS_2D_Lookup_Table
      settings: SourceProductName=PACCAR Technical Center MBDS Library
      settings: AttributesFormatString=|
      | Row Axis: TCM_NCRS_SHIFT_UP_GEARNUM_STEP_MPV (1)
      | Column Axis: TCM_NCRS_SHIFT_UP_THROTTLE_STEP_MPV (%)
      | Data Axis: TCM_NCRS_SHIFT_UP_DATA_MPV (rpm)
      | Interpolation Method: Linear
  Add1 : Sum  Inputs=+++
  Constant : PTC_MBDS_LIB/Extras/Sources/Constant  Value2=TCM_NUMBER_OF_GEARS_APV  PTC_MBDS_BlockVersion=5.41  PTC_BlockType=PTC_MBDS_Constant
      settings: SourceProductName=PACCAR Technical Center MBDS Library
      settings: AttributesFormatString=|
      | Value: 12
      | Unit: '1'
  Constant3 : Constant  Value=0  OutDataTypeStr=boolean
  Logical Operator : Logic  AllPortsSameDT=off  OutDataTypeStr=boolean
  Logical Operator1 : Logic  Operator=NOT  AllPortsSameDT=off  OutDataTypeStr=boolean
  Relational Operator : RelationalOperator  Operator=>  OutDataTypeStr=boolean  RndMeth=Nearest
  Relational Operator1 : RelationalOperator  Operator=<  OutDataTypeStr=boolean  RndMeth=Nearest
  Switch2 : Switch  Criteria=u2 ~= 0
  UpShift_F : Outport
  wires:
  PrevGearIn/1 -> Relational Operator1/1
  PedalPosition/1 -> 2D_Lookup_Table/2
  GradeOffset/1 -> Add1/3
  2D_Lookup_Table/1 -> Add1/2
  Add1/1 -> Relational Operator/2
  Switch2/1 -> UpShift_F/1
  GearCurrent/1 -> 2D_Lookup_Table/1
  Relational Operator/1 -> Switch2/1
  Constant/1 -> Relational Operator1/2  "TCM_NUMBER_OF_GEARS_APV"
  Constant3/1 -> Switch2/3
  Logical Operator/1 -> Switch2/2
  HoldState/1 -> Logical Operator1/1
  Relational Operator1/1 -> Logical Operator/2
  Logical Operator1/1 -> Logical Operator/1
  EngineSpeedRPM/1 -> Relational Operator/1
  EngineBrakeOffset/1 -> Add1/1

== system SUB_ECU_Transmission/TCM/NeutralCoast/OffDelayTimer/S-R Reset Priority ==
  R : Inport
  S : Inport  Port=2
  Logic : CombinatorialLogic  TruthTable=[0;1;0;0;1;1;0;0]
  Memory : Memory  InheritSampleTime=on
  Mux : Mux  Inputs=3
  Q : Outport  InitialOutput=0
  wires:
  R/1 -> Mux/2
  S/1 -> Mux/1
  Memory/1 -> Mux/3
  Logic/1 -> Q/1, Memory/1
  Mux/1 -> Logic/1

== system SUB_ECU_Transmission/TCM/NeutralCoast/OffDelayTimer/S-R Set Priority ==
  S : Inport
  R : Inport  Port=2
  Logic : CombinatorialLogic  TruthTable=[0;1;0;0;1;1;1;1]
  Memory : Memory  InheritSampleTime=on
  Mux : Mux  Inputs=3
  Q : Outport  InitialOutput=0
  wires:
  Mux/1 -> Logic/1
  Logic/1 -> Memory/1, Q/1
  Memory/1 -> Mux/3
  S/1 -> Mux/1
  R/1 -> Mux/2

== system SUB_ECU_Transmission/TCM/ShiftTableGear/RetDemDownshift/meters_to_rev_per_km ==
  In : Inport
  Constant4 : PTC_MBDS_LIB/Extras/Sources/Constant  Value2=1  PTC_MBDS_BlockVersion=5.41  PTC_BlockType=PTC_MBDS_Constant
      settings: SourceProductName=PACCAR Technical Center MBDS Library
  Divide2 : Product  Inputs=*/  OutDataTypeStr=Inherit: Inherit via back propagation  SaturateOnIntegerOverflow=on  InputSameDT=on
      settings: AttributesFormatString=Saturate: %<SaturateOnIntegerOverflow>
  Gain : Gain  Gain=pi * 0.001
  Out1 : Outport
  wires:
  Divide2/1 -> Out1/1
  In/1 -> Gain/1
  Gain/1 -> Divide2/2
  Constant4/1 -> Divide2/1

== stateflow chart SUB_ECU_Transmission/TCM/ShiftControlChart ==
  state CutTorque
    en: State = 2;
    en: OCME = 3;
    en: OCMR = 3;
    en: TrqReqE = DrvDemTrq;
    en: TrqReqR = RetDrv;
    du: TrqReqE = TrqReqE - TrqRampRate * TimeStep;
    du: TrqReqE = max(TrqReqE, 0);
    du: TrqReqR = TrqReqR - TrqRampRate * TimeStep;
    du: TrqReqR = max(TrqReqR, 0);
  state OpenClutch
    en: State = 3;
    en: MainClutchClose = false;
    en: TrqReqE = 0;
    en: TrqReqR = 0;
  state RevForShift
    en: State = 4;
    en: Timer1 = 0;
    en: OCME = 2;
    en: OCMR = 3;
    en: TrqReqE = 0.7;
    en: TrqReqR = 0;
    en: EspdEntry = EngSpd;
    en: EspdError = 0;
    du: Timer1 = Timer1 + TimeStep;
    du: EspdError = EngSpd - EspdEntry;
  state RevHigherForSkipShift
    en: State = 5;
    en: Timer1 = 0;
    en: OCME = 2;
    en: OCMR = 3;
    en: TrqReqE = 0.8;
    en: TrqReqR = 0;
    en: EspdEntry = EngSpd;
    en: EspdError = 0;
    du: Timer1 = Timer1 + TimeStep;
    du: EspdError = EngSpd - EspdEntry;
  state Init
    en: State = 1;
    en: MainClutchClose = false;
    en: GearNumber = 0;
    en: OCME = 0;
    en: OCMR = 0;
    en: TrqReqE = 0;
    en: TrqReqR = 0;
  state ChangeGear
    State = 6;
    OCME = 3;
    OCMR = 3;
    TrqReqE = 0;
    TrqReqR = 0;
  state UpShift
    State = 7;
    GearNumber = GearNumber + GearIncr;
  state DownShift
    State = 8;
    GearNumber = GearNumber - GearIncr;
  state CloseClutch
    State = 9;
    MainClutchClose = true;
  state Delay
    en: State = 10;
    en: Timer1 = 0;
    du: Timer1 = Timer1 + TimeStep;
  state RampUpRetarderTorque
    en: State = 11;
    du: TrqReqR = TrqReqR + ...
    TrqRampRate * TimeStep;
    du: TrqReqR = min(TrqReqR, RetDrv);
  state RampUpEngineTorque
    en: State = 12;
    du: TrqReqE = TrqReqE + ...
    TrqRampRate * TimeStep;
    du: TrqReqE = min(TrqReqE, DrvDemTrq);
  state ShiftComplete
    en: State = 13;
    en: TimerAntiHunt = 0;
    en: OCME = 0;
    en: OCMR = 0;
    en: TrqReqE = 0;
    en: TrqReqR = 0;
    du: TimerAntiHunt = TimerAntiHunt + TimeStep;
  (junction 46) -> CutTorque
  (junction 125) -> (junction 46)
  CutTorque -> OpenClutch : [(TrqReqE < 0.03) && (TrqReqR < 0.03)]
  OpenClutch -> (junction 134) [order 1] : [(TransmissionStateLock == 2) &&( GearIncr > 1) && DownShift]
  (junction 134) -> RevHigherForSkipShift
  OpenClutch -> ChangeGear [order 3] : [TransmissionStateLock == 2]
  OpenClutch -> RevForShift [order 2] : [(TransmissionStateLock == 2) && DownShift]
  (default) -> Init
  RevForShift -> ChangeGear : [(EspdError >= 385) || (Timer1 > 3)]
  RevHigherForSkipShift -> (junction 132) : [(EspdError >= 770) || (Timer1 > 3)]
  Init -> ChangeGear [order 1] : [(PRND == 3) && DownShift]
      | {LatchDownShift = true;
      | LatchUpShift = false;}
  (junction 132) -> ChangeGear
  Init -> ChangeGear [order 2] : [(PRND == 3) && UpShift]
      | {LatchUpShift = true;
      | LatchDownShift = false;}
  ChangeGear -> UpShift [order 2] : [LatchUpShift && ~DownShift]
  ChangeGear -> CloseClutch [order 3]
  ChangeGear -> DownShift [order 1] : [LatchDownShift && ~UpShift]
  (junction 127) -> Init
  UpShift -> CloseClutch
  DownShift -> CloseClutch
  CloseClutch -> Delay
  Delay -> (junction 146) [order 1] : [(Timer1 >= ShiftDelay) && ...
      | (TransmissionStateLock == 5) && ...
      | (DrvDemTrq > 0) && ...
      | (DrvDemTrq >= RetDrv)]
  (junction 146) -> RampUpEngineTorque
  Delay -> ShiftComplete [order 3] : [(Timer1 >= ShiftDelay) && ...
      |    (TransmissionStateLock == 5)]
  Delay -> RampUpRetarderTorque [order 2] : [(Timer1 >= ShiftDelay) && ...
      | (TransmissionStateLock == 5) && ...
      | (RetDrv > 0)]
  RampUpRetarderTorque -> ShiftComplete : [TrqReqR > (RetDrv - 0.03)]
  RampUpEngineTorque -> (junction 149) : [TrqReqE > (DrvDemTrq - 0.03)]
  ShiftComplete -> (junction 127) [order 1] : [PRND ~= 3]
  ShiftComplete -> (junction 125) [order 2] : [(TimerAntiHunt > AntiHuntDelay) && DownShift]
      | {LatchDownShift = true;
      | LatchUpShift = false;}
  (junction 149) -> ShiftComplete
  (junction 136) -> (junction 125)
  ShiftComplete -> (junction 136) [order 3] : [(TimerAntiHunt > AntiHuntDelay) && UpShift]
      | {LatchUpShift = true;
      | LatchDownShift = false;}
  data: MainClutchClose output boolean; UpShift input boolean; DownShift input boolean; GearIncr input double; DrvDemTrq input; RetDrv input; EngSpd input; PRND input; VehSpd input; TransmissionStateLock input; LatchUpShift local boolean; LatchDownShift local boolean; TimerAntiHunt local double; AntiHuntDelay input double; TimeStep input double; Timer1 local double; TrqRampRate input; ShiftDelay input; EspdEntry local; EspdError local; OCME output; TrqReqE output; OCMR output; TrqReqR output; State output size=1; GearNumber output

== stateflow chart SUB_ECU_Transmission/TCM/NeutralCoast/Chart ==
  state init
    entry:State=0;
  state Delay
    entry:State=4;
    entry:Timer1=0;
    during:Timer1=Timer1+TimeStep;
  state Enabled
    entry:State=1;
  state CheckSpeedAccel
    entry:State=5;
  state CheckSpeedDeccel
    entry:State=6;
  state TimeDelay
    entry:State=2;
    during:Timer1=Timer1+TimeStep;
  state Coasting
    entry:State=3;
    en:CoastingActive=1;
  (default) -> init
  Coasting -> init [order 1] : [!Enable]
      | {CoastingActive=0;}
  Enabled -> init [order 1] : [!Enable]
  TimeDelay -> init [order 1] : [!Enable]
  init -> Enabled : [Enable]
  Delay -> Enabled : [Timer1>=0]
  Enabled -> (junction 39) [order 2] : [VehAccelerationCondition&&...
      | !BrakingActive&&...
      | ActTrqPer<CoastActTrqLowThr&&...
      | !ShiftInProcess]
  (junction 24) -> Delay [order 1] : [!VehSpeedCondition||...
      | !VehAccelerationCondition||...
      | BrakingActive||....
      | AccelPedPos>=CoastPedUpThr]...
      | {CoastingActive=0;}
  (junction 39) -> CheckSpeedAccel [order 2]
  (junction 39) -> CheckSpeedDeccel [order 1] : [VehAccel<0&&...
      | !BrakingActivePrev]
  CheckSpeedAccel -> TimeDelay : [VehicleSpd<(CruiseControlSetSpd+MaxVehSpdThr-3)]
  CheckSpeedDeccel -> TimeDelay : [VehicleSpd>(CruiseControlSetSpd+MinVehSpdThr+3)]
  TimeDelay -> (junction 24) [order 2] : [Timer1>=0]
  Coasting -> (junction 24) [order 2]
  (junction 24) -> Coasting [order 2]
  data: Enable input double; VehicleSpd input double; CruiseControlSetSpd input double; VehSpeedCondition input boolean; VehAccelerationCondition input boolean; BrakingActive input boolean; AccelPedPos input double; ActTrqPer input double; ShiftInProcess input double; VehAccel input double; CoastActTrqUpThr input double; CoastActTrqLowThr input double; CoastingActive output double; State output double; CoastPedUpThr input double; CoastPedLowThr input double; TimeStep input double; Timer1 local double; MaxVehSpdThr input double; MinVehSpdThr input double; BrakingActivePrev input boolean
